simulink library "hydlib"  (Simulink 6.0)
settings: Solver=ode45  SolverMode=SingleTasking  StartTime=0.0  StopTime=10.0  RelTol=1e-3
values from neighbouring files (symbols this model uses):
  M = (lenHouse*widHouse*htHouse+tan(pitRoof)*widHouse*lenHouse)*densAir    [thermdat.m]
undefined symbols (not defined in the file or in its folder): Ac, beta, C1, C2, Cd, I, K, L, p30, Qmax, rho, sgn, V30
libraries: hydlib x2
settings Model: Creator=The MathWorks Inc.  LastModifiedBy=batserve  ExtModeAutoUpdateStatusClock=off
settings OptimizationCC: BooleanDataType=off
settings DebuggingCC: CheckExecutionContextPreStartOutputMsg=on  CheckExecutionContextRuntimeOutputMsg=on  SolverPrmCheckMsg=none
settings HardwareCC: TargetUnknown=on

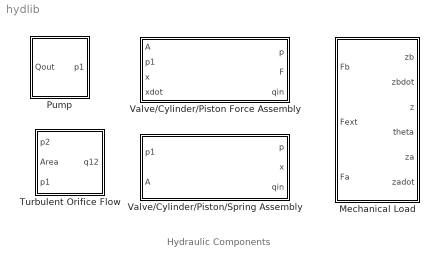
== system hydlib ==
  note: Hydraulic Components
  Mechanical Load : Subsystem  PropExecContextAcrossSSBoundary=on  mask(Rod){L=L, M=M, I=I}
      mask prompts: L "Length:"; M "Mass at center of rotation:"; I "Moment of inertia:"
      mask help: This block models a rigid rod subject to forces Fa and Fb at either end and Fext at its center. The outputs z, za and zb represent linear displacement and theta is the angle of rotation.
      mask Help: See "Using Simulink and Stateflow in Automotive Applications" for a mathematical derivation of the subsystem operation.  Contact your MathWorks distributor to obtain a copy.
      mask Display: plot(-25,-8,100,108,[40 50 60 50 40],[10 10 90 90 10], [0 40], [10 10], [30 40 30], [8 10 12], [40 50 40], [88 90 92], [0 50], [90 90], [15 45], [49 49], [15 45], [51 51], [20 10 20], [48 50 52], 50*ones(2,10), [0:10:90; 5:10:95])
  Pump : Subsystem  PropExecContextAcrossSSBoundary=on  mask(Pump){t=[0        .04     .04     .05    .05     .1], Qpump=Qmax*[1 1 0 0 1 1], p10=Qmax/C2*2, C2=C2}
      mask prompts: t "Time:"; Qpump "Pump flow:"; p10 "Initial pressure:"; C2 "Leakage flow gain:"
      mask help: The pump model provides a supply pressure for a hydraulic system. The gross flow, Qpump, is split between the supply flow demand (load), Qout, and leakage, Qleak. The Time and Pump flow vectors entered below specify Qpump and the leakage flow gain determines Qleak = C2*p1, where p1 is the supply pressure.
      mask init:
      | T = t';
      | Q = Qpump';
      mask Help: See "Using Simulink and Stateflow in Automotive Applications" for a mathematical derivation of the subsystem operation.  Contact your MathWorks distributor to obtain a copy.
      mask Display: plot(cos(0:0.1:2*pi),sin(0:0.1:2*pi), [0.5 1 0.5 0.5],[-0.3 0 0.3 -0.3])
  Turbulent Orifice Flow : Subsystem  PropExecContextAcrossSSBoundary=on
      mask Help: See "Using Simulink and Stateflow in Automotive Applications" for a mathematical derivation of the subsystem operation.  Contact your MathWorks distributor to obtain a copy.
      mask Display:
      | plot(-0.75,-1.25,0.75,1.25,[0 0],[1 -1],0.5*cos(-pi/4:.1:pi/4)-0.55, 0.5*sin(-pi/4:.1:pi/4),-0.5*cos(-pi/4:.1:pi/4)+0.55, 0.5*sin(-pi/4:.1:pi/4));
      | plot([-0.4, 0.4], [-0.4, 0.4], [0.3, 0.4], [0.4, 0.4], [0.37 0.4], [0.25, 0.4])
  Valve/Cylinder/Piston Force Assembly : Subsystem  PropExecContextAcrossSSBoundary=on  mask(ValveCylinderPistonForceAssy){C1=C1, Ac=Ac, Cd=Cd, rho=rho, V30=V30, beta=beta, p30=p30}
      mask prompts: C1 "Flow gain from valve to actuator:"; Ac "Actuator cross-sectional area:"; Cd "Discharge coefficient:"; rho "Fluid density:"; V30 "Cylinder volume at x = 0:"; beta "Bulk modulus:"; p30 "Initial pressure:"
      mask help:
      | A hydraulic cylinder is fed through a variable-area control valve, producing an axial piston force.
      |
      | inputs                                              outputs
      | A = valve flow area                         p = valve and piston pressure vector
      | p1 = supply pressure                       F = piston force
      | x = load (piston) position                 qin = input flow rate
      | xdot = load (piston) velocity
      |
      | see "Using Simulink and Stateflow in Automotive Applications" for a mathematical derivation of the subsystem operation
      mask Help: See "Using Simulink and Stateflow in Automotive Applications" for a mathematical derivation of the subsystem operation.  Contact your MathWorks distributor to obtain a copy.
      mask Display: plot(0,30,200,70,[180,94,140,140,180,94,94,94,10],[40,40,40,60,60,60,50,50,50],[94,94],[50,40]);plot(50+50*cos(-0.6*pi:0.05:-0.4*pi),101+50*sin(-0.6*pi:0.05:-0.4*pi));plot(50+50*cos(-0.6*pi:0.05:-0.4*pi),-1-50*sin(-0.6*pi:0.05:-0.4*pi),[40,60],[45 55],[50,60,60],[53 55 53.],[140,150;160,170;180,190]',[50;50]*ones(1,3))
  Valve/Cylinder/Piston/Spring Assembly : Subsystem  PropExecContextAcrossSSBoundary=on  mask(Valve/Cylinder/Piston/Spring Assembly){K=K, C1=C1, Ac=Ac, Cd=Cd, rho=rho, V30=V30, beta=beta}
      mask prompts: K "Spring rate:"; C1 "Flow gain from valve to actuator:"; Ac "Actuator cross-sectional area:"; Cd "Discharge coefficient:"; rho "Fluid density:"; V30 "Cylinder volume at x = 0:"; beta "Bulk modulus:"
      mask help:
      | A hydraulic cylinder is fed through a variable-area control valve, producing an axial piston force which compresses a linear spring.
      |
      | inputs                                              outputs
      | A = valve flow area                         p = valve and piston pressure vector
      | p1 = supply pressure                       x = piston displacement
      |                                                        qin = input flow rate
      |
      | see "Using Simulink and Stateflow in Automotive Applications" for a mathematical derivation of the subsystem operation.
      mask Help: See "Using Simulink and Stateflow in Automotive Applications" for a mathematical derivation of the subsystem operation.  Contact your MathWorks distributor to obtain a copy.
      mask Display: plot(0,30,210,70,[180,94,140,140,180,94,94,94,10],[40,40,40,60,60,60,50,50,50],[94,94],[50,40]);plot(50+50*cos(-0.6*pi:0.05:-0.4*pi),101+50*sin(-0.6*pi:0.05:-0.4*pi));plot(50+50*cos(-0.6*pi:0.05:-0.4*pi),-1-50*sin(-0.6*pi:0.05:-0.4*pi),[40,60],[45 55],[50,60,60],[53 55 53.],[140,150;160,170;180,190]',[50;50]*ones(1,3), [180 180], [60 55], [180 180], [40 45], 143.5+3.5*cos(0:.1:6.28), 57.5+2*sin(0:.1:6.28),143.5+3.5*cos(0:.1:6.28), 42.5+2*sin(0:.1:6.28),176.5+3.5*cos(0:.1:6.28), 57.5+2*sin(0:.1:6.28),176.5+3.5*cos(0:.1:6.28), 42.5+2*sin(0:.1:6.28),160+3.5*cos(0:.1:6.28), 57.5+2*sin(0:.1:6.28),160+3.5*cos(0:.1:6.28),42.5+2*sin(0:.1:6.28))

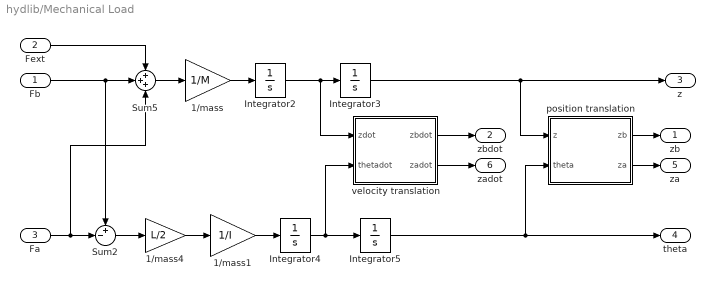
== system hydlib/Mechanical Load ==
  Fb : Inport  Port=1  LatchInput=off
  Fext : Inport  Port=2  LatchInput=off
  Fa : Inport  Port=3  LatchInput=off
  1/mass : Gain  Gain=1/M  SaturateOnIntegerOverflow=on
  1/mass1 : Gain  Gain=1/I  SaturateOnIntegerOverflow=on
  1/mass4 : Gain  Gain=L/2  SaturateOnIntegerOverflow=on
  Integrator{2..5} (4 alike) : Integrator  UpperSaturationLimit=Inf  LowerSaturationLimit=-Inf
  Sum2 : Sum  Inputs=+-|  SaturateOnIntegerOverflow=on  InputSameDT=on
  Sum5 : Sum  Inputs=+++  SaturateOnIntegerOverflow=on  InputSameDT=on
  position translation : Subsystem  PropExecContextAcrossSSBoundary=on
  velocity translation : Subsystem  PropExecContextAcrossSSBoundary=on
  zb : Outport  InitialOutput=0
  zbdot : Outport  Port=2  InitialOutput=0
  z : Outport  Port=3  InitialOutput=0
  theta : Outport  Port=4  InitialOutput=0
  za : Outport  Port=5  InitialOutput=0
  zadot : Outport  Port=6  InitialOutput=0
  wires:
  Fb/1 -> Sum5/2, Sum2/1
  Sum5/1 -> 1/mass/1
  Integrator2/1 -> velocity translation/1(zdot), Integrator3/1
  1/mass/1 -> Integrator2/1
  Integrator3/1 -> position translation/1(z), z/1
  position translation/1(zb) -> zb/1
  position translation/2(za) -> za/1
  velocity translation/2(zadot) -> zadot/1
  velocity translation/1(zbdot) -> zbdot/1
  Integrator5/1 -> position translation/2(theta), theta/1
  Fa/1 -> Sum5/3, Sum2/2
  1/mass1/1 -> Integrator4/1
  Integrator4/1 -> velocity translation/2(thetadot), Integrator5/1
  1/mass4/1 -> 1/mass1/1
  Sum2/1 -> 1/mass4/1
  Fext/1 -> Sum5/1

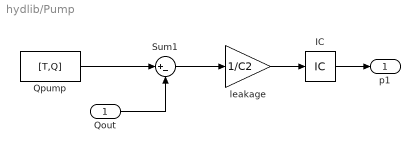
== system hydlib/Pump ==
  Qout : Inport  Port=1  LatchInput=off
  IC : InitialCondition  Value=p10
  Qpump : FromWorkspace  VariableName=[T,Q]  SampleTime=0
  Sum1 : Sum  Inputs=|+-  SaturateOnIntegerOverflow=on  InputSameDT=on
  leakage : Gain  Gain=1/C2  SaturateOnIntegerOverflow=on
  p1 : Outport  InitialOutput=0
  wires:
  Qpump/1 -> Sum1/1
  Sum1/1 -> leakage/1
  Qout/1 -> Sum1/2
  leakage/1 -> IC/1
  IC/1 -> p1/1

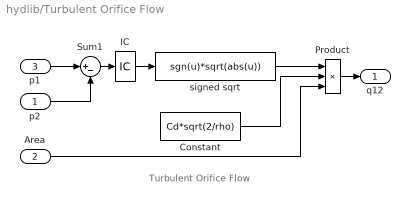
== system hydlib/Turbulent Orifice Flow ==
  note: Turbulent Orifice Flow
  p2 : Inport  Port=1  LatchInput=off
  Area : Inport  Port=2  LatchInput=off
  p1 : Inport  Port=3  LatchInput=off
  Constant : Constant  Value=Cd*sqrt(2/rho)
  IC : InitialCondition  Value=0
  Product : Product  Inputs=3  SaturateOnIntegerOverflow=on  RndMeth=Zero  InputSameDT=on
  Sum1 : Sum  Inputs=|+-  SaturateOnIntegerOverflow=on  InputSameDT=on
  signed sqrt : Fcn  Expr=sgn(u)*sqrt(abs(u))
  q12 : Outport  InitialOutput=0
  wires:
  p2/1 -> Sum1/2
  p1/1 -> Sum1/1
  Area/1 -> Product/3
  Product/1 -> q12/1
  signed sqrt/1 -> Product/1
  Constant/1 -> Product/2
  Sum1/1 -> IC/1
  IC/1 -> signed sqrt/1

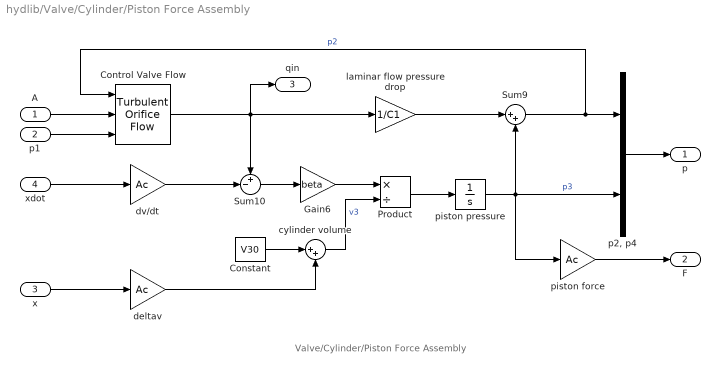
== system hydlib/Valve/Cylinder/Piston Force Assembly ==
  note: Valve/Cylinder/Piston Force Assembly
  A : Inport  Port=1  LatchInput=off
  p1 : Inport  Port=2  LatchInput=off
  x : Inport  Port=3  LatchInput=off
  xdot : Inport  Port=4  LatchInput=off
  Constant : Constant  Value=V30
  Control Valve Flow : hydlib/Turbulent Orifice Flow
  Gain6 : Gain  Gain=beta  SaturateOnIntegerOverflow=on
  Product : Product  Inputs=*/  SaturateOnIntegerOverflow=on  RndMeth=Zero  InputSameDT=on
  Sum10 : Sum  Inputs=+-|  SaturateOnIntegerOverflow=on  InputSameDT=on
  Sum9 : Sum  Inputs=|++  SaturateOnIntegerOverflow=on  InputSameDT=on
  cylinder volume : Sum  Inputs=|++  SaturateOnIntegerOverflow=on  InputSameDT=on
  deltav : Gain  Gain=Ac  SaturateOnIntegerOverflow=on
  dv/dt : Gain  Gain=Ac  SaturateOnIntegerOverflow=on
  laminar flow pressure drop : Gain  Gain=1/C1  SaturateOnIntegerOverflow=on
  "p2, p4" : Mux  Inputs=2
  piston force : Gain  Gain=Ac  SaturateOnIntegerOverflow=on
  piston pressure : Integrator  InitialCondition=p30  LimitOutput=on  LowerSaturationLimit=0
  p : Outport  InitialOutput=0
  F : Outport  Port=2  InitialOutput=0
  qin : Outport  Port=3  InitialOutput=0
  wires:
  piston force/1 -> F/1
  p1/1 -> Control Valve Flow/3
  Sum9/1 -> "p2, p4"/1, Control Valve Flow/1  "p2"
  laminar flow pressure drop/1 -> Sum9/1
  A/1 -> Control Valve Flow/2
  "p2, p4"/1 -> p/1
  Control Valve Flow/1 -> laminar flow pressure drop/1, Sum10/1, qin/1
  Product/1 -> piston pressure/1
  Gain6/1 -> Product/1
  cylinder volume/1 -> Product/2  "v3"
  piston pressure/1 -> Sum9/2, "p2, p4"/2, piston force/1  "p3"
  xdot/1 -> dv/dt/1
  dv/dt/1 -> Sum10/2
  Sum10/1 -> Gain6/1
  Constant/1 -> cylinder volume/1
  deltav/1 -> cylinder volume/2
  x/1 -> deltav/1

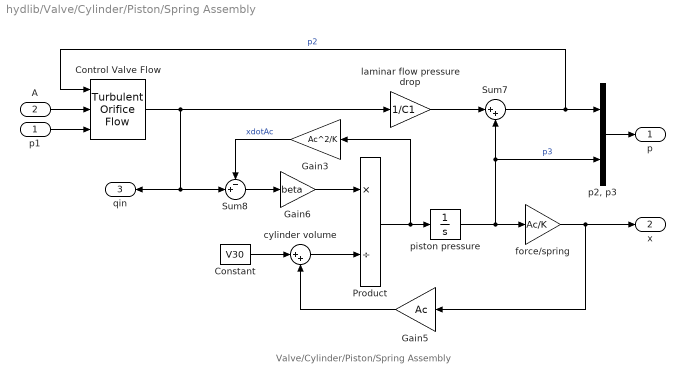
== system hydlib/Valve/Cylinder/Piston/Spring Assembly ==
  note: Valve/Cylinder/Piston/Spring Assembly
  p1 : Inport  Port=1  LatchInput=off
  A : Inport  Port=2  LatchInput=off
  Constant : Constant  Value=V30
  Control Valve Flow : hydlib/Turbulent Orifice Flow
  Gain3 : Gain  Orientation=left  Gain=Ac^2/K  SaturateOnIntegerOverflow=on
  Gain5 : Gain  Orientation=left  Gain=Ac  SaturateOnIntegerOverflow=on
  Gain6 : Gain  Gain=beta  SaturateOnIntegerOverflow=on
  Product : Product  Inputs=*/  SaturateOnIntegerOverflow=on  RndMeth=Zero  InputSameDT=on
  Sum7 : Sum  Inputs=|++  SaturateOnIntegerOverflow=on  InputSameDT=on
  Sum8 : Sum  Inputs=-+|  SaturateOnIntegerOverflow=on  InputSameDT=on
  cylinder volume : Sum  Inputs=|++  SaturateOnIntegerOverflow=on  InputSameDT=on
  force/spring : Gain  Gain=Ac/K  SaturateOnIntegerOverflow=on
  laminar flow pressure drop : Gain  Gain=1/C1  SaturateOnIntegerOverflow=on
  "p2, p3" : Mux  Inputs=2
  piston pressure : Integrator  LimitOutput=on  LowerSaturationLimit=0
  p : Outport  InitialOutput=0
  x : Outport  Port=2  InitialOutput=0
  qin : Outport  Orientation=left  Port=3  InitialOutput=0
  wires:
  Constant/1 -> cylinder volume/1
  Gain3/1 -> Sum8/1  "xdotAc"
  p1/1 -> Control Valve Flow/3
  Sum7/1 -> "p2, p3"/1, Control Valve Flow/1  "p2"
  laminar flow pressure drop/1 -> Sum7/1
  Control Valve Flow/1 -> Sum8/2, qin/1, laminar flow pressure drop/1
  A/1 -> Control Valve Flow/2
  "p2, p3"/1 -> p/1
  Sum8/1 -> Gain6/1
  Gain5/1 -> cylinder volume/2
  Gain6/1 -> Product/1
  Product/1 -> piston pressure/1, Gain3/1
  cylinder volume/1 -> Product/2
  force/spring/1 -> Gain5/1, x/1
  piston pressure/1 -> Sum7/2, "p2, p3"/2, force/spring/1  "p3"

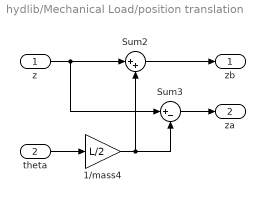
== system hydlib/Mechanical Load/position translation ==
  z : Inport  Port=1  LatchInput=off
  theta : Inport  Port=2  LatchInput=off
  1/mass4 : Gain  Gain=L/2  SaturateOnIntegerOverflow=on
  Sum2 : Sum  Inputs=|++  SaturateOnIntegerOverflow=on  InputSameDT=on
  Sum3 : Sum  Inputs=|+-  SaturateOnIntegerOverflow=on  InputSameDT=on
  zb : Outport  InitialOutput=0
  za : Outport  Port=2  InitialOutput=0
  wires:
  Sum3/1 -> za/1
  Sum2/1 -> zb/1
  z/1 -> Sum3/1, Sum2/1
  1/mass4/1 -> Sum3/2, Sum2/2
  theta/1 -> 1/mass4/1

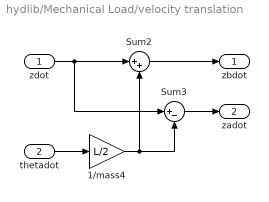
== system hydlib/Mechanical Load/velocity translation ==
  zdot : Inport  Port=1  LatchInput=off
  thetadot : Inport  Port=2  LatchInput=off
  1/mass4 : Gain  Gain=L/2  SaturateOnIntegerOverflow=on
  Sum2 : Sum  Inputs=|++  SaturateOnIntegerOverflow=on  InputSameDT=on
  Sum3 : Sum  Inputs=|+-  SaturateOnIntegerOverflow=on  InputSameDT=on
  zbdot : Outport  InitialOutput=0
  zadot : Outport  Port=2  InitialOutput=0
  wires:
  Sum3/1 -> zadot/1
  Sum2/1 -> zbdot/1
  zdot/1 -> Sum2/1, Sum3/1
  1/mass4/1 -> Sum2/2, Sum3/2
  thetadot/1 -> 1/mass4/1
